simulink model "Project_Simulink"  (R2024a)
settings: Solver=ode45  StartTime=0.0  StopTime=20  MaxStep=1e-3  RelTol=1e-3
settings Model: Creator=Chand  LastModifiedBy=Chand
settings DebuggingCC: UnderSpecifiedDimensionMsg=warning

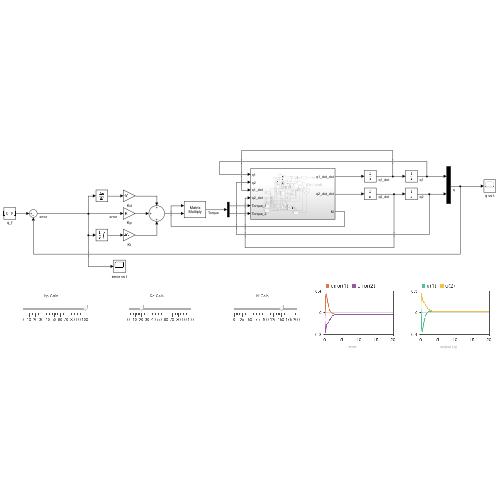
[thumbnail: Simulink's stored preview of the top-level diagram]
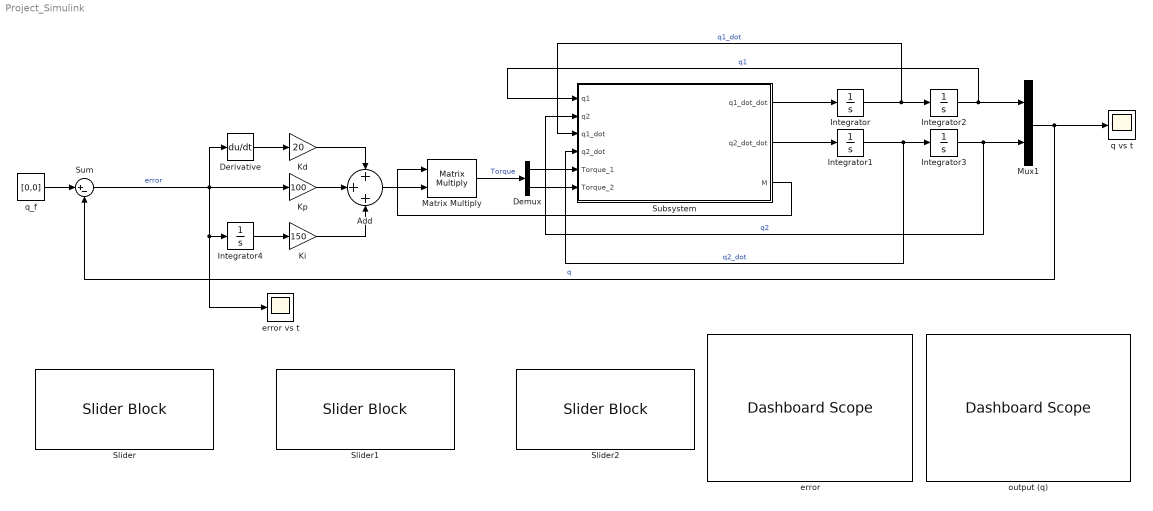
== system Project_Simulink ==
  Add : Sum  Inputs=+++
  Demux : Demux  Outputs=2
  Derivative : Derivative
  Integrator : Integrator
  Integrator1 : Integrator
  Integrator2 : Integrator  InitialCondition=0.1
  Integrator3 : Integrator  InitialCondition=0.1
  Integrator4 : Integrator  LimitOutput=on  UpperSaturationLimit=20  LowerSaturationLimit=-20
  Kd : Gain  Gain=20
  Ki : Gain  Gain=150
  Kp : Gain  Gain=100
  Matrix Multiply : Product  Multiplication=Matrix(*)
  Mux1 : Mux  Inputs=2
  Slider : SliderBlock
  Slider1 : SliderBlock
  Slider2 : SliderBlock  ScaleMax=200
  Subsystem : Subsystem
  Sum : Sum  Inputs=|+-
  error : DashboardScope
  error vs t : Scope
  output (q) : DashboardScope
  q vs t : Scope
  q_f : Constant  Value=[0,0]
  wires:
  Subsystem/1(q1_dot_dot) -> Integrator/1
  Subsystem/2(q2_dot_dot) -> Integrator1/1
  Integrator2/1 -> Subsystem/1(q1), Mux1/1  "q1"
  Integrator/1 -> Integrator2/1, Subsystem/3(q1_dot)  "q1_dot"
  Integrator1/1 -> Subsystem/4(q2_dot), Integrator3/1  "q2_dot"
  Demux/1 -> Subsystem/5(Torque_1)
  Integrator3/1 -> Subsystem/2(q2), Mux1/2  "q2"
  Demux/2 -> Subsystem/6(Torque_2)
  Derivative/1 -> Kd/1
  Sum/1 -> Integrator4/1, error vs t/1, Derivative/1, Kp/1  "error"
  Integrator4/1 -> Ki/1
  Kp/1 -> Add/2
  Kd/1 -> Add/1
  Ki/1 -> Add/3
  Mux1/1 -> q vs t/1, Sum/2  "q"
  q_f/1 -> Sum/1
  Add/1 -> Matrix Multiply/2
  Matrix Multiply/1 -> Demux/1  "Torque"
  Subsystem/3(M) -> Matrix Multiply/1

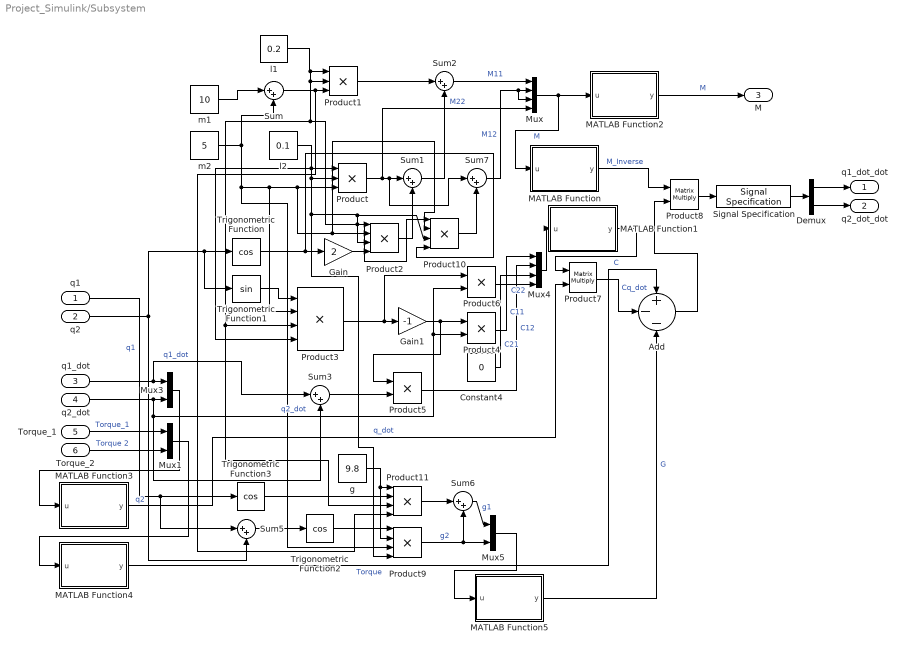
== system Project_Simulink/Subsystem ==
  q1 : Inport
  q2 : Inport  Port=2
  q1_dot : Inport  Port=3
  q2_dot : Inport  Port=4
  Torque_1 : Inport  Port=5
  Torque_2 : Inport  Port=6
  Add : Sum  Inputs=+--
  Constant4 : Constant  Value=0
  Demux : Demux  Outputs=2
  Gain : Gain  Gain=2
  Gain1 : Gain  Gain=-1
  MATLAB Function : MATLAB Function  TreatAsAtomicUnit=on
  MATLAB Function1 : MATLAB Function  TreatAsAtomicUnit=on
  MATLAB Function2 : MATLAB Function  TreatAsAtomicUnit=on
  MATLAB Function3 : MATLAB Function  TreatAsAtomicUnit=on
  MATLAB Function4 : MATLAB Function  TreatAsAtomicUnit=on
  MATLAB Function5 : MATLAB Function  TreatAsAtomicUnit=on
  Mux : Mux
  Mux1 : Mux  Inputs=2
  Mux3 : Mux  Inputs=2
  Mux4 : Mux
  Mux5 : Mux  Inputs=2
  Product : Product  Inputs=3
  Product1 : Product  Inputs=3
  Product{2..3,9..11} (5 alike) : Product  Inputs=4
  Product4 : Product
  Product5 : Product
  Product6 : Product
  Product7 : Product  Multiplication=Matrix(*)
  Product8 : Product  Multiplication=Matrix(*)
  Signal Specification : SignalSpecification  Dimensions=[2 1]
  Sum{,1..3,5..7} (7 alike) : Sum  Inputs=|++
  Trigonometric Function : Trigonometry  Operator=cos
  Trigonometric Function1 : Trigonometry
  Trigonometric Function2 : Trigonometry  Operator=cos
  Trigonometric Function3 : Trigonometry  Operator=cos
  g : Constant  Value=9.8
  l1 : Constant  Value=0.2
  l2 : Constant  Value=0.1
  m1 : Constant  Value=10
  m2 : Constant  Value=5
  q1_dot_dot : Outport
  q2_dot_dot : Outport  Port=2
  M : Outport  Port=3
  wires:
  q2/1 -> Sum5/2, Trigonometric Function1/1, Trigonometric Function/1  "q2"
  l2/1 -> Product9/4, Product2/3, Product10/3, Product/2, Product/1, Product3/4
  m1/1 -> Sum/1
  Sum/1 -> Product11/4, Product1/3
  l1/1 -> Product3/3, Product11/3, Product10/1, Product2/1, Product1/2, Product1/1
  Trigonometric Function/1 -> Gain/1, Product10/4
  Product/1 -> Mux/4, Sum7/1, Sum1/1  "M22"
  Product1/1 -> Sum2/1
  Sum1/1 -> Sum2/2
  Sum2/1 -> Mux/1  "M11"
  Product2/1 -> Sum1/2
  m2/1 -> Product2/2, Product10/2, Product/3, Product3/2, Product9/3, Sum/2
  Gain/1 -> Product2/4
  Torque_1/1 -> Mux1/1  "Torque_1"
  Torque_2/1 -> Mux1/2  "Torque 2"
  q2_dot/1 -> Sum3/2, Product4/2, Product6/2, Mux3/2  "q2_dot"
  q1_dot/1 -> Sum3/1, Mux3/1  "q1_dot"
  q1/1 -> Sum5/1, Trigonometric Function3/1  "q1"
  Trigonometric Function1/1 -> Product3/1
  Product3/1 -> Product6/1, Gain1/1
  Sum3/1 -> Product5/2
  Gain1/1 -> Product4/1, Product5/1
  Product6/1 -> Mux4/4  "C22"
  Product5/1 -> Mux4/2  "C12"
  Product4/1 -> Mux4/1  "C11"
  Constant4/1 -> Mux4/3  "C21"
  Product7/1 -> Add/2  "Cq_dot"
  Add/1 -> Product8/2
  Demux/1 -> q1_dot_dot/1
  Demux/2 -> q2_dot_dot/1
  Sum5/1 -> Trigonometric Function2/1
  Trigonometric Function2/1 -> Product9/1
  g/1 -> Product9/2, Product11/1
  Product9/1 -> Sum6/2, Mux5/2  "g2"
  MATLAB Function5/1(y) -> Add/3  "G"
  Sum6/1 -> Mux5/1  "g1"
  Product11/1 -> Sum6/1
  Trigonometric Function3/1 -> Product11/2
  Mux/1 -> MATLAB Function2/1(u), MATLAB Function/1(u)  "M"
  Mux4/1 -> MATLAB Function1/1(u)
  MATLAB Function1/1(y) -> Product7/1  "C"
  Mux3/1 -> MATLAB Function3/1(u)
  MATLAB Function3/1(y) -> Product7/2  "q_dot"
  Mux1/1 -> MATLAB Function4/1(u)
  MATLAB Function4/1(y) -> Add/1  "Torque"
  Mux5/1 -> MATLAB Function5/1(u)
  Product8/1 -> Signal Specification/1
  Signal Specification/1 -> Demux/1
  MATLAB Function/1(y) -> Product8/1  "M_Inverse"
  Product10/1 -> Sum7/2
  Sum7/1 -> Mux/3, Mux/2  "M12"
  MATLAB Function2/1(y) -> M/1  "M"

== matlab function Project_Simulink/Subsystem/MATLAB Function ==
  data: u input; y output
function y = fcn(u)
    mat=[u(1),u(2);
        u(3),u(4)];
    y=inv(mat);
end

== matlab function Project_Simulink/Subsystem/MATLAB Function2 ==
  data: u input; y output
function y = fcn(u)
    y=[u(1),u(2);
        u(3),u(4)];
end

== matlab function Project_Simulink/Subsystem/MATLAB Function3 ==
  data: u input; y output
function y = fcn(u)
    y=[u(1);u(2)];
end

== matlab function Project_Simulink/Subsystem/MATLAB Function4 ==
  data: u input; y output
function y = fcn(u)
    y=[u(1);u(2)];
end

== matlab function Project_Simulink/Subsystem/MATLAB Function5 ==
  data: u input; y output
function y = fcn(u)
    y=[u(1);u(2)];
end

== matlab function Project_Simulink/Subsystem/MATLAB Function1 ==
  data: u input; y output
function y = fcn(u)
    y=[u(1),u(2);
       u(3),u(4)];
end
